simulink model "NewKitchen_REB_workstation"  (R2020b)
settings: Solver=FixedStepAuto  StartTime=sim_start  StopTime=sim_end  FixedStep=sim_interval  RelTol=1e-3
undefined symbols (not defined in the file): AmbientTem, Power1, Power2, Power3, Velocity1, Velocity2
libraries: dspswit3 x6
(part 2 of 3)

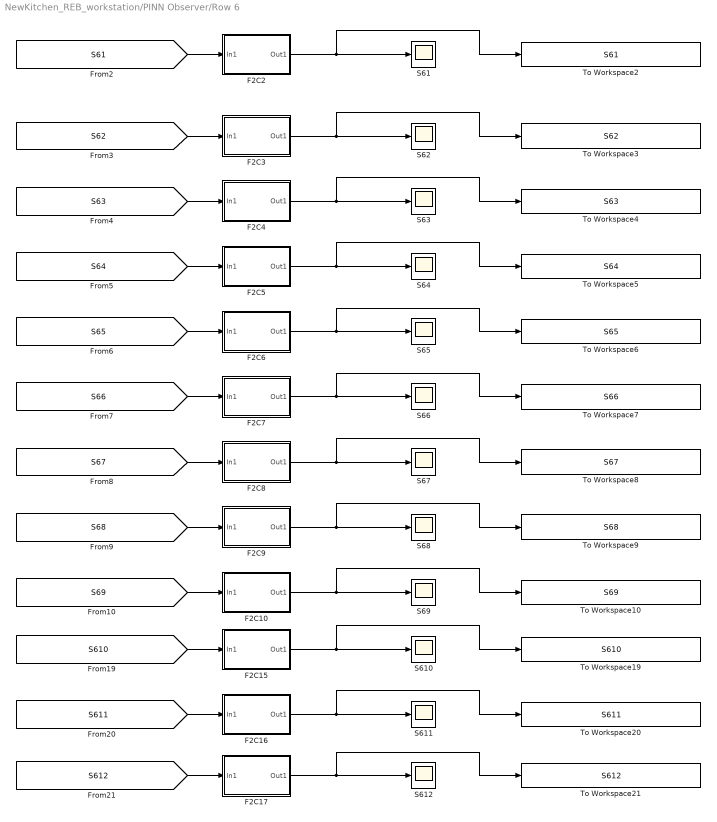
== system NewKitchen_REB_workstation/PINN Observer/Row 6 ==
  F2C10 : Subsystem
  F2C15 : Subsystem
  F2C16 : Subsystem
  F2C17 : Subsystem
  F2C2 : Subsystem
  F2C3 : Subsystem
  F2C4 : Subsystem
  F2C5 : Subsystem
  F2C6 : Subsystem
  F2C7 : Subsystem
  F2C8 : Subsystem
  F2C9 : Subsystem
  S{61..69,610..612} (12 alike) : Scope
  To Workspace10 : ToWorkspace  VariableName=S69  SampleTime=-1
  To Workspace19 : ToWorkspace  VariableName=S610  SampleTime=-1
  To Workspace2 : ToWorkspace  VariableName=S61  SampleTime=-1
  To Workspace20 : ToWorkspace  VariableName=S611  SampleTime=-1
  To Workspace21 : ToWorkspace  VariableName=S612  SampleTime=-1
  To Workspace3 : ToWorkspace  VariableName=S62  SampleTime=-1
  To Workspace4 : ToWorkspace  VariableName=S63  SampleTime=-1
  To Workspace5 : ToWorkspace  VariableName=S64  SampleTime=-1
  To Workspace6 : ToWorkspace  VariableName=S65  SampleTime=-1
  To Workspace7 : ToWorkspace  VariableName=S66  SampleTime=-1
  To Workspace8 : ToWorkspace  VariableName=S67  SampleTime=-1
  To Workspace9 : ToWorkspace  VariableName=S68  SampleTime=-1
  wires:
  [S64] -> F2C5/1(In1)
  [S62] -> F2C3/1(In1)
  [S63] -> F2C4/1(In1)
  F2C8/1(Out1) -> To Workspace8/1, S67/1
  F2C3/1(Out1) -> S62/1, To Workspace3/1
  F2C2/1(Out1) -> To Workspace2/1, S61/1
  [S61] -> F2C2/1(In1)
  F2C15/1(Out1) -> S610/1, To Workspace19/1
  [S68] -> F2C9/1(In1)
  [S611] -> F2C16/1(In1)
  F2C10/1(Out1) -> To Workspace10/1, S69/1
  F2C16/1(Out1) -> To Workspace20/1, S611/1
  F2C6/1(Out1) -> To Workspace6/1, S65/1
  [S610] -> F2C15/1(In1)
  F2C9/1(Out1) -> S68/1, To Workspace9/1
  [S66] -> F2C7/1(In1)
  F2C5/1(Out1) -> S64/1, To Workspace5/1
  F2C4/1(Out1) -> To Workspace4/1, S63/1
  [S612] -> F2C17/1(In1)
  [S65] -> F2C6/1(In1)
  F2C17/1(Out1) -> S612/1, To Workspace21/1
  F2C7/1(Out1) -> S66/1, To Workspace7/1
  [S69] -> F2C10/1(In1)
  [S67] -> F2C8/1(In1)

== system NewKitchen_REB_workstation/PINN Observer/Row 7 ==
  F2C10 : Subsystem
  F2C15 : Subsystem
  F2C16 : Subsystem
  F2C17 : Subsystem
  F2C2 : Subsystem
  F2C3 : Subsystem
  F2C4 : Subsystem
  F2C5 : Subsystem
  F2C6 : Subsystem
  F2C7 : Subsystem
  F2C8 : Subsystem
  F2C9 : Subsystem
  S{71..79,710..712} (12 alike) : Scope
  To Workspace10 : ToWorkspace  VariableName=S79  SampleTime=-1
  To Workspace19 : ToWorkspace  VariableName=S710  SampleTime=-1
  To Workspace2 : ToWorkspace  VariableName=S71  SampleTime=-1
  To Workspace20 : ToWorkspace  VariableName=S711  SampleTime=-1
  To Workspace21 : ToWorkspace  VariableName=S712  SampleTime=-1
  To Workspace3 : ToWorkspace  VariableName=S72  SampleTime=-1
  To Workspace4 : ToWorkspace  VariableName=S73  SampleTime=-1
  To Workspace5 : ToWorkspace  VariableName=S74  SampleTime=-1
  To Workspace6 : ToWorkspace  VariableName=S75  SampleTime=-1
  To Workspace7 : ToWorkspace  VariableName=S76  SampleTime=-1
  To Workspace8 : ToWorkspace  VariableName=S77  SampleTime=-1
  To Workspace9 : ToWorkspace  VariableName=S78  SampleTime=-1
  wires:
  [S77] -> F2C8/1(In1)
  [S79] -> F2C10/1(In1)
  F2C7/1(Out1) -> To Workspace7/1, S76/1
  F2C17/1(Out1) -> To Workspace21/1, S712/1
  [S75] -> F2C6/1(In1)
  [S712] -> F2C17/1(In1)
  F2C4/1(Out1) -> S73/1, To Workspace4/1
  F2C5/1(Out1) -> To Workspace5/1, S74/1
  [S76] -> F2C7/1(In1)
  F2C9/1(Out1) -> To Workspace9/1, S78/1
  [S710] -> F2C15/1(In1)
  F2C6/1(Out1) -> S75/1, To Workspace6/1
  F2C16/1(Out1) -> S711/1, To Workspace20/1
  F2C10/1(Out1) -> S79/1, To Workspace10/1
  [S711] -> F2C16/1(In1)
  [S78] -> F2C9/1(In1)
  F2C15/1(Out1) -> To Workspace19/1, S710/1
  [S71] -> F2C2/1(In1)
  F2C2/1(Out1) -> S71/1, To Workspace2/1
  F2C3/1(Out1) -> To Workspace3/1, S72/1
  F2C8/1(Out1) -> S77/1, To Workspace8/1
  [S73] -> F2C4/1(In1)
  [S72] -> F2C3/1(In1)
  [S74] -> F2C5/1(In1)

== system NewKitchen_REB_workstation/PINN Observer/Row 8 ==
  F2C10 : Subsystem
  F2C15 : Subsystem
  F2C16 : Subsystem
  F2C17 : Subsystem
  F2C2 : Subsystem
  F2C3 : Subsystem
  F2C4 : Subsystem
  F2C5 : Subsystem
  F2C6 : Subsystem
  F2C7 : Subsystem
  F2C8 : Subsystem
  F2C9 : Subsystem
  S{81..89,810..812} (12 alike) : Scope
  To Workspace10 : ToWorkspace  VariableName=S89  SampleTime=-1
  To Workspace19 : ToWorkspace  VariableName=S810  SampleTime=-1
  To Workspace2 : ToWorkspace  VariableName=S81  SampleTime=-1
  To Workspace20 : ToWorkspace  VariableName=S811  SampleTime=-1
  To Workspace21 : ToWorkspace  VariableName=S812  SampleTime=-1
  To Workspace3 : ToWorkspace  VariableName=S82  SampleTime=-1
  To Workspace4 : ToWorkspace  VariableName=S83  SampleTime=-1
  To Workspace5 : ToWorkspace  VariableName=S84  SampleTime=-1
  To Workspace6 : ToWorkspace  VariableName=S85  SampleTime=-1
  To Workspace7 : ToWorkspace  VariableName=S86  SampleTime=-1
  To Workspace8 : ToWorkspace  VariableName=S87  SampleTime=-1
  To Workspace9 : ToWorkspace  VariableName=S88  SampleTime=-1
  wires:
  [S84] -> F2C5/1(In1)
  [S82] -> F2C3/1(In1)
  [S83] -> F2C4/1(In1)
  F2C8/1(Out1) -> To Workspace8/1, S87/1
  F2C3/1(Out1) -> S82/1, To Workspace3/1
  F2C2/1(Out1) -> To Workspace2/1, S81/1
  [S81] -> F2C2/1(In1)
  F2C15/1(Out1) -> S810/1, To Workspace19/1
  [S88] -> F2C9/1(In1)
  [S811] -> F2C16/1(In1)
  F2C10/1(Out1) -> To Workspace10/1, S89/1
  F2C16/1(Out1) -> To Workspace20/1, S811/1
  F2C6/1(Out1) -> To Workspace6/1, S85/1
  [S810] -> F2C15/1(In1)
  F2C9/1(Out1) -> S88/1, To Workspace9/1
  [S86] -> F2C7/1(In1)
  F2C5/1(Out1) -> S84/1, To Workspace5/1
  F2C4/1(Out1) -> To Workspace4/1, S83/1
  [S812] -> F2C17/1(In1)
  [S85] -> F2C6/1(In1)
  F2C17/1(Out1) -> S812/1, To Workspace21/1
  F2C7/1(Out1) -> S86/1, To Workspace7/1
  [S89] -> F2C10/1(In1)
  [S87] -> F2C8/1(In1)

== system NewKitchen_REB_workstation/PINN Observer/Row 9 ==
  F2C10 : Subsystem
  F2C15 : Subsystem
  F2C16 : Subsystem
  F2C17 : Subsystem
  F2C2 : Subsystem
  F2C3 : Subsystem
  F2C4 : Subsystem
  F2C5 : Subsystem
  F2C6 : Subsystem
  F2C7 : Subsystem
  F2C8 : Subsystem
  F2C9 : Subsystem
  S{91..99,910..912} (12 alike) : Scope
  To Workspace10 : ToWorkspace  VariableName=S99  SampleTime=-1
  To Workspace19 : ToWorkspace  VariableName=S910  SampleTime=-1
  To Workspace2 : ToWorkspace  VariableName=S91  SampleTime=-1
  To Workspace20 : ToWorkspace  VariableName=S911  SampleTime=-1
  To Workspace21 : ToWorkspace  VariableName=S912  SampleTime=-1
  To Workspace3 : ToWorkspace  VariableName=S92  SampleTime=-1
  To Workspace4 : ToWorkspace  VariableName=S93  SampleTime=-1
  To Workspace5 : ToWorkspace  VariableName=S94  SampleTime=-1
  To Workspace6 : ToWorkspace  VariableName=S95  SampleTime=-1
  To Workspace7 : ToWorkspace  VariableName=S96  SampleTime=-1
  To Workspace8 : ToWorkspace  VariableName=S97  SampleTime=-1
  To Workspace9 : ToWorkspace  VariableName=S98  SampleTime=-1
  wires:
  [S97] -> F2C8/1(In1)
  [S99] -> F2C10/1(In1)
  F2C7/1(Out1) -> To Workspace7/1, S96/1
  F2C17/1(Out1) -> To Workspace21/1, S912/1
  [S95] -> F2C6/1(In1)
  [S912] -> F2C17/1(In1)
  F2C4/1(Out1) -> S93/1, To Workspace4/1
  F2C5/1(Out1) -> To Workspace5/1, S94/1
  [S96] -> F2C7/1(In1)
  F2C9/1(Out1) -> To Workspace9/1, S98/1
  [S910] -> F2C15/1(In1)
  F2C6/1(Out1) -> S95/1, To Workspace6/1
  F2C16/1(Out1) -> S911/1, To Workspace20/1
  F2C10/1(Out1) -> S99/1, To Workspace10/1
  [S911] -> F2C16/1(In1)
  [S98] -> F2C9/1(In1)
  F2C15/1(Out1) -> To Workspace19/1, S910/1
  [S91] -> F2C2/1(In1)
  F2C2/1(Out1) -> S91/1, To Workspace2/1
  F2C3/1(Out1) -> To Workspace3/1, S92/1
  F2C8/1(Out1) -> S97/1, To Workspace8/1
  [S93] -> F2C4/1(In1)
  [S92] -> F2C3/1(In1)
  [S94] -> F2C5/1(In1)

== system NewKitchen_REB_workstation/Signals/AmbientTem ==
  1-D Lookup Table : Lookup_n-D  NumberOfTableDimensions=1  BreakpointsForDimension1=AmbientTem(:,1)  Table=AmbientTem(:,2)  InterpMethod=Flat  InternalRulePriority=Speed  RndMeth=Simplest  InputSameDT=on
  Counter : dspswit3/Counter  Direction=Up  CountEvent=Free running  CounterSize=User defined  MaxCount=480  InitialCount=1  Output=Count  HitValue=1  ResetInput=off  SamplesPerFrame=1  Ts=60  CntDtype=double  HitDtype=Logical
  MATLAB Function : MATLAB Function  Commented=on  TreatAsAtomicUnit=on
  signal : Outport
  wires:
  Counter/1 -> 1-D Lookup Table/1
  1-D Lookup Table/1 -> signal/1

== system NewKitchen_REB_workstation/Signals/C2F3 ==
  signal : Inport
  Constant : Constant  Value=273.15
  Subtract : Sum
  Tout : Outport
  wires:
  signal/1 -> Subtract/1
  Constant/1 -> Subtract/2
  Subtract/1 -> Tout/1

== system NewKitchen_REB_workstation/Signals/Power1 ==
  1-D Lookup Table : Lookup_n-D  NumberOfTableDimensions=1  BreakpointsForDimension1=Power1(:,1)  Table=Power1(:,2)  InterpMethod=Flat  InternalRulePriority=Speed  RndMeth=Simplest  InputSameDT=on
  Counter : dspswit3/Counter  Direction=Up  CountEvent=Free running  CounterSize=User defined  MaxCount=480  InitialCount=1  Output=Count  HitValue=1  ResetInput=off  SamplesPerFrame=1  Ts=60  CntDtype=double  HitDtype=Logical
  MATLAB Function : MATLAB Function  Commented=on  TreatAsAtomicUnit=on
  P1 : Outport
  wires:
  Counter/1 -> 1-D Lookup Table/1
  1-D Lookup Table/1 -> P1/1

== system NewKitchen_REB_workstation/Signals/Power2 ==
  1-D Lookup Table : Lookup_n-D  NumberOfTableDimensions=1  BreakpointsForDimension1=Power2(:,1)  Table=Power2(:,2)  InterpMethod=Flat  InternalRulePriority=Speed  RndMeth=Simplest  InputSameDT=on
  Counter : dspswit3/Counter  Direction=Up  CountEvent=Free running  CounterSize=User defined  MaxCount=480  InitialCount=1  Output=Count  HitValue=1  ResetInput=off  SamplesPerFrame=1  Ts=60  CntDtype=double  HitDtype=Logical
  MATLAB Function : MATLAB Function  Commented=on  TreatAsAtomicUnit=on
  P2 : Outport
  wires:
  Counter/1 -> 1-D Lookup Table/1
  1-D Lookup Table/1 -> P2/1

== system NewKitchen_REB_workstation/Signals/Power3 ==
  1-D Lookup Table : Lookup_n-D  NumberOfTableDimensions=1  BreakpointsForDimension1=Power3(:,1)  Table=Power3(:,2)  InterpMethod=Flat  InternalRulePriority=Speed  RndMeth=Simplest  InputSameDT=on
  Counter : dspswit3/Counter  Direction=Up  CountEvent=Free running  CounterSize=User defined  MaxCount=480  InitialCount=1  Output=Count  HitValue=1  ResetInput=off  SamplesPerFrame=1  Ts=60  CntDtype=double  HitDtype=Logical
  MATLAB Function : MATLAB Function  Commented=on  TreatAsAtomicUnit=on
  P3 : Outport
  wires:
  Counter/1 -> 1-D Lookup Table/1
  1-D Lookup Table/1 -> P3/1

== system NewKitchen_REB_workstation/Signals/V1 ==
  1-D Lookup Table : Lookup_n-D  NumberOfTableDimensions=1  BreakpointsForDimension1=Velocity1(:,1)  Table=Velocity1(:,2)  InterpMethod=Flat  InternalRulePriority=Speed  RndMeth=Simplest  InputSameDT=on
  Counter : dspswit3/Counter  Direction=Up  CountEvent=Free running  CounterSize=User defined  MaxCount=480  InitialCount=1  Output=Count  HitValue=1  ResetInput=off  SamplesPerFrame=1  Ts=60  CntDtype=double  HitDtype=Logical
  MATLAB Function : MATLAB Function  Commented=on  TreatAsAtomicUnit=on
  V1 : Outport
  wires:
  Counter/1 -> 1-D Lookup Table/1
  1-D Lookup Table/1 -> V1/1

== system NewKitchen_REB_workstation/Signals/V2 ==
  1-D Lookup Table : Lookup_n-D  NumberOfTableDimensions=1  BreakpointsForDimension1=Velocity2(:,1)  Table=Velocity2(:,2)  InterpMethod=Flat  InternalRulePriority=Speed  RndMeth=Simplest  InputSameDT=on
  Counter : dspswit3/Counter  Direction=Up  CountEvent=Free running  CounterSize=User defined  MaxCount=480  InitialCount=1  Output=Count  HitValue=1  ResetInput=off  SamplesPerFrame=1  Ts=60  CntDtype=double  HitDtype=Logical
  MATLAB Function : MATLAB Function  Commented=on  TreatAsAtomicUnit=on
  V2 : Outport
  wires:
  Counter/1 -> 1-D Lookup Table/1
  1-D Lookup Table/1 -> V2/1

== system NewKitchen_REB_workstation/PINN Observer/Boundary Four/F2C10 ==
  In1 : Inport
  Constant : Constant  Value=273.15
  Subtract : Sum  Inputs=+-
  Out1 : Outport
  wires:
  In1/1 -> Subtract/1
  Constant/1 -> Subtract/2
  Subtract/1 -> Out1/1

== system NewKitchen_REB_workstation/PINN Observer/Boundary Four/F2C15 ==
  In1 : Inport
  Constant : Constant  Value=273.15
  Subtract : Sum  Inputs=+-
  Out1 : Outport
  wires:
  Subtract/1 -> Out1/1
  Constant/1 -> Subtract/2
  In1/1 -> Subtract/1

== system NewKitchen_REB_workstation/PINN Observer/Boundary Four/F2C16 ==
  In1 : Inport
  Constant : Constant  Value=273.15
  Subtract : Sum  Inputs=+-
  Out1 : Outport
  wires:
  In1/1 -> Subtract/1
  Constant/1 -> Subtract/2
  Subtract/1 -> Out1/1

== system NewKitchen_REB_workstation/PINN Observer/Boundary Four/F2C17 ==
  In1 : Inport
  Constant : Constant  Value=273.15
  Subtract : Sum  Inputs=+-
  Out1 : Outport
  wires:
  Subtract/1 -> Out1/1
  Constant/1 -> Subtract/2
  In1/1 -> Subtract/1

== system NewKitchen_REB_workstation/PINN Observer/Boundary Four/F2C18 ==
  In1 : Inport
  Constant : Constant  Value=273.15
  Subtract : Sum  Inputs=+-
  Out1 : Outport
  wires:
  In1/1 -> Subtract/1
  Constant/1 -> Subtract/2
  Subtract/1 -> Out1/1

== system NewKitchen_REB_workstation/PINN Observer/Boundary Four/F2C19 ==
  In1 : Inport
  Constant : Constant  Value=273.15
  Subtract : Sum  Inputs=+-
  Out1 : Outport
  wires:
  Subtract/1 -> Out1/1
  Constant/1 -> Subtract/2
  In1/1 -> Subtract/1

== system NewKitchen_REB_workstation/PINN Observer/Boundary Four/F2C2 ==
  In1 : Inport
  Constant : Constant  Value=273.15
  Subtract : Sum  Inputs=+-
  Out1 : Outport
  wires:
  In1/1 -> Subtract/1
  Constant/1 -> Subtract/2
  Subtract/1 -> Out1/1

== system NewKitchen_REB_workstation/PINN Observer/Boundary Four/F2C3 ==
  In1 : Inport
  Constant : Constant  Value=273.15
  Subtract : Sum  Inputs=+-
  Out1 : Outport
  wires:
  Subtract/1 -> Out1/1
  Constant/1 -> Subtract/2
  In1/1 -> Subtract/1

== system NewKitchen_REB_workstation/PINN Observer/Boundary Four/F2C4 ==
  In1 : Inport
  Constant : Constant  Value=273.15
  Subtract : Sum  Inputs=+-
  Out1 : Outport
  wires:
  In1/1 -> Subtract/1
  Constant/1 -> Subtract/2
  Subtract/1 -> Out1/1

== system NewKitchen_REB_workstation/PINN Observer/Boundary Four/F2C5 ==
  In1 : Inport
  Constant : Constant  Value=273.15
  Subtract : Sum  Inputs=+-
  Out1 : Outport
  wires:
  Subtract/1 -> Out1/1
  Constant/1 -> Subtract/2
  In1/1 -> Subtract/1

== system NewKitchen_REB_workstation/PINN Observer/Boundary Four/F2C6 ==
  In1 : Inport
  Constant : Constant  Value=273.15
  Subtract : Sum  Inputs=+-
  Out1 : Outport
  wires:
  In1/1 -> Subtract/1
  Constant/1 -> Subtract/2
  Subtract/1 -> Out1/1

== system NewKitchen_REB_workstation/PINN Observer/Boundary Four/F2C7 ==
  In1 : Inport
  Constant : Constant  Value=273.15
  Subtract : Sum  Inputs=+-
  Out1 : Outport
  wires:
  Subtract/1 -> Out1/1
  Constant/1 -> Subtract/2
  In1/1 -> Subtract/1

== system NewKitchen_REB_workstation/PINN Observer/Boundary Four/F2C8 ==
  In1 : Inport
  Constant : Constant  Value=273.15
  Subtract : Sum  Inputs=+-
  Out1 : Outport
  wires:
  In1/1 -> Subtract/1
  Constant/1 -> Subtract/2
  Subtract/1 -> Out1/1

== system NewKitchen_REB_workstation/PINN Observer/Boundary Four/F2C9 ==
  In1 : Inport
  Constant : Constant  Value=273.15
  Subtract : Sum  Inputs=+-
  Out1 : Outport
  wires:
  Subtract/1 -> Out1/1
  Constant/1 -> Subtract/2
  In1/1 -> Subtract/1

== system NewKitchen_REB_workstation/PINN Observer/Boundary One/F2C10 ==
  In1 : Inport
  Constant : Constant  Value=273.15
  Subtract : Sum  Inputs=+-
  Out1 : Outport
  wires:
  Subtract/1 -> Out1/1
  Constant/1 -> Subtract/2
  In1/1 -> Subtract/1

== system NewKitchen_REB_workstation/PINN Observer/Boundary One/F2C15 ==
  In1 : Inport
  Constant : Constant  Value=273.15
  Subtract : Sum  Inputs=+-
  Out1 : Outport
  wires:
  In1/1 -> Subtract/1
  Constant/1 -> Subtract/2
  Subtract/1 -> Out1/1

== system NewKitchen_REB_workstation/PINN Observer/Boundary One/F2C16 ==
  In1 : Inport
  Constant : Constant  Value=273.15
  Subtract : Sum  Inputs=+-
  Out1 : Outport
  wires:
  Subtract/1 -> Out1/1
  Constant/1 -> Subtract/2
  In1/1 -> Subtract/1

== system NewKitchen_REB_workstation/PINN Observer/Boundary One/F2C17 ==
  In1 : Inport
  Constant : Constant  Value=273.15
  Subtract : Sum  Inputs=+-
  Out1 : Outport
  wires:
  In1/1 -> Subtract/1
  Constant/1 -> Subtract/2
  Subtract/1 -> Out1/1

== system NewKitchen_REB_workstation/PINN Observer/Boundary One/F2C18 ==
  In1 : Inport
  Constant : Constant  Value=273.15
  Subtract : Sum  Inputs=+-
  Out1 : Outport
  wires:
  Subtract/1 -> Out1/1
  Constant/1 -> Subtract/2
  In1/1 -> Subtract/1

== system NewKitchen_REB_workstation/PINN Observer/Boundary One/F2C19 ==
  In1 : Inport
  Constant : Constant  Value=273.15
  Subtract : Sum  Inputs=+-
  Out1 : Outport
  wires:
  In1/1 -> Subtract/1
  Constant/1 -> Subtract/2
  Subtract/1 -> Out1/1

== system NewKitchen_REB_workstation/PINN Observer/Boundary One/F2C2 ==
  In1 : Inport
  Constant : Constant  Value=273.15
  Subtract : Sum  Inputs=+-
  Out1 : Outport
  wires:
  Subtract/1 -> Out1/1
  Constant/1 -> Subtract/2
  In1/1 -> Subtract/1

== system NewKitchen_REB_workstation/PINN Observer/Boundary One/F2C3 ==
  In1 : Inport
  Constant : Constant  Value=273.15
  Subtract : Sum  Inputs=+-
  Out1 : Outport
  wires:
  In1/1 -> Subtract/1
  Constant/1 -> Subtract/2
  Subtract/1 -> Out1/1

== system NewKitchen_REB_workstation/PINN Observer/Boundary One/F2C4 ==
  In1 : Inport
  Constant : Constant  Value=273.15
  Subtract : Sum  Inputs=+-
  Out1 : Outport
  wires:
  Subtract/1 -> Out1/1
  Constant/1 -> Subtract/2
  In1/1 -> Subtract/1

== system NewKitchen_REB_workstation/PINN Observer/Boundary One/F2C5 ==
  In1 : Inport
  Constant : Constant  Value=273.15
  Subtract : Sum  Inputs=+-
  Out1 : Outport
  wires:
  In1/1 -> Subtract/1
  Constant/1 -> Subtract/2
  Subtract/1 -> Out1/1

== system NewKitchen_REB_workstation/PINN Observer/Boundary One/F2C6 ==
  In1 : Inport
  Constant : Constant  Value=273.15
  Subtract : Sum  Inputs=+-
  Out1 : Outport
  wires:
  Subtract/1 -> Out1/1
  Constant/1 -> Subtract/2
  In1/1 -> Subtract/1

== system NewKitchen_REB_workstation/PINN Observer/Boundary One/F2C7 ==
  In1 : Inport
  Constant : Constant  Value=273.15
  Subtract : Sum  Inputs=+-
  Out1 : Outport
  wires:
  In1/1 -> Subtract/1
  Constant/1 -> Subtract/2
  Subtract/1 -> Out1/1

== system NewKitchen_REB_workstation/PINN Observer/Boundary One/F2C8 ==
  In1 : Inport
  Constant : Constant  Value=273.15
  Subtract : Sum  Inputs=+-
  Out1 : Outport
  wires:
  Subtract/1 -> Out1/1
  Constant/1 -> Subtract/2
  In1/1 -> Subtract/1

== system NewKitchen_REB_workstation/PINN Observer/Boundary One/F2C9 ==
  In1 : Inport
  Constant : Constant  Value=273.15
  Subtract : Sum  Inputs=+-
  Out1 : Outport
  wires:
  In1/1 -> Subtract/1
  Constant/1 -> Subtract/2
  Subtract/1 -> Out1/1

== system NewKitchen_REB_workstation/PINN Observer/Boundary Three/F2C10 ==
  In1 : Inport
  Constant : Constant  Value=273.15
  Subtract : Sum  Inputs=+-
  Out1 : Outport
  wires:
  Subtract/1 -> Out1/1
  Constant/1 -> Subtract/2
  In1/1 -> Subtract/1

== system NewKitchen_REB_workstation/PINN Observer/Boundary Three/F2C2 ==
  In1 : Inport
  Constant : Constant  Value=273.15
  Subtract : Sum  Inputs=+-
  Out1 : Outport
  wires:
  Subtract/1 -> Out1/1
  Constant/1 -> Subtract/2
  In1/1 -> Subtract/1

== system NewKitchen_REB_workstation/PINN Observer/Boundary Three/F2C3 ==
  In1 : Inport
  Constant : Constant  Value=273.15
  Subtract : Sum  Inputs=+-
  Out1 : Outport
  wires:
  In1/1 -> Subtract/1
  Constant/1 -> Subtract/2
  Subtract/1 -> Out1/1

== system NewKitchen_REB_workstation/PINN Observer/Boundary Three/F2C4 ==
  In1 : Inport
  Constant : Constant  Value=273.15
  Subtract : Sum  Inputs=+-
  Out1 : Outport
  wires:
  Subtract/1 -> Out1/1
  Constant/1 -> Subtract/2
  In1/1 -> Subtract/1

== system NewKitchen_REB_workstation/PINN Observer/Boundary Three/F2C5 ==
  In1 : Inport
  Constant : Constant  Value=273.15
  Subtract : Sum  Inputs=+-
  Out1 : Outport
  wires:
  In1/1 -> Subtract/1
  Constant/1 -> Subtract/2
  Subtract/1 -> Out1/1

== system NewKitchen_REB_workstation/PINN Observer/Boundary Three/F2C6 ==
  In1 : Inport
  Constant : Constant  Value=273.15
  Subtract : Sum  Inputs=+-
  Out1 : Outport
  wires:
  Subtract/1 -> Out1/1
  Constant/1 -> Subtract/2
  In1/1 -> Subtract/1

== system NewKitchen_REB_workstation/PINN Observer/Boundary Three/F2C7 ==
  In1 : Inport
  Constant : Constant  Value=273.15
  Subtract : Sum  Inputs=+-
  Out1 : Outport
  wires:
  In1/1 -> Subtract/1
  Constant/1 -> Subtract/2
  Subtract/1 -> Out1/1

== system NewKitchen_REB_workstation/PINN Observer/Boundary Three/F2C8 ==
  In1 : Inport
  Constant : Constant  Value=273.15
  Subtract : Sum  Inputs=+-
  Out1 : Outport
  wires:
  Subtract/1 -> Out1/1
  Constant/1 -> Subtract/2
  In1/1 -> Subtract/1

== system NewKitchen_REB_workstation/PINN Observer/Boundary Three/F2C9 ==
  In1 : Inport
  Constant : Constant  Value=273.15
  Subtract : Sum  Inputs=+-
  Out1 : Outport
  wires:
  In1/1 -> Subtract/1
  Constant/1 -> Subtract/2
  Subtract/1 -> Out1/1

== system NewKitchen_REB_workstation/PINN Observer/Boundary Two/F2C10 ==
  In1 : Inport
  Constant : Constant  Value=273.15
  Subtract : Sum  Inputs=+-
  Out1 : Outport
  wires:
  In1/1 -> Subtract/1
  Constant/1 -> Subtract/2
  Subtract/1 -> Out1/1

== system NewKitchen_REB_workstation/PINN Observer/Boundary Two/F2C2 ==
  In1 : Inport
  Constant : Constant  Value=273.15
  Subtract : Sum  Inputs=+-
  Out1 : Outport
  wires:
  In1/1 -> Subtract/1
  Constant/1 -> Subtract/2
  Subtract/1 -> Out1/1

== system NewKitchen_REB_workstation/PINN Observer/Boundary Two/F2C3 ==
  In1 : Inport
  Constant : Constant  Value=273.15
  Subtract : Sum  Inputs=+-
  Out1 : Outport
  wires:
  Subtract/1 -> Out1/1
  Constant/1 -> Subtract/2
  In1/1 -> Subtract/1

== system NewKitchen_REB_workstation/PINN Observer/Boundary Two/F2C4 ==
  In1 : Inport
  Constant : Constant  Value=273.15
  Subtract : Sum  Inputs=+-
  Out1 : Outport
  wires:
  In1/1 -> Subtract/1
  Constant/1 -> Subtract/2
  Subtract/1 -> Out1/1

== system NewKitchen_REB_workstation/PINN Observer/Boundary Two/F2C5 ==
  In1 : Inport
  Constant : Constant  Value=273.15
  Subtract : Sum  Inputs=+-
  Out1 : Outport
  wires:
  Subtract/1 -> Out1/1
  Constant/1 -> Subtract/2
  In1/1 -> Subtract/1

== system NewKitchen_REB_workstation/PINN Observer/Boundary Two/F2C6 ==
  In1 : Inport
  Constant : Constant  Value=273.15
  Subtract : Sum  Inputs=+-
  Out1 : Outport
  wires:
  In1/1 -> Subtract/1
  Constant/1 -> Subtract/2
  Subtract/1 -> Out1/1

== system NewKitchen_REB_workstation/PINN Observer/Boundary Two/F2C7 ==
  In1 : Inport
  Constant : Constant  Value=273.15
  Subtract : Sum  Inputs=+-
  Out1 : Outport
  wires:
  Subtract/1 -> Out1/1
  Constant/1 -> Subtract/2
  In1/1 -> Subtract/1

== system NewKitchen_REB_workstation/PINN Observer/Boundary Two/F2C8 ==
  In1 : Inport
  Constant : Constant  Value=273.15
  Subtract : Sum  Inputs=+-
  Out1 : Outport
  wires:
  In1/1 -> Subtract/1
  Constant/1 -> Subtract/2
  Subtract/1 -> Out1/1

== system NewKitchen_REB_workstation/PINN Observer/Boundary Two/F2C9 ==
  In1 : Inport
  Constant : Constant  Value=273.15
  Subtract : Sum  Inputs=+-
  Out1 : Outport
  wires:
  Subtract/1 -> Out1/1
  Constant/1 -> Subtract/2
  In1/1 -> Subtract/1

== system NewKitchen_REB_workstation/PINN Observer/Row 1/F2C10 ==
  In1 : Inport
  Constant : Constant  Value=273.15
  Subtract : Sum  Inputs=+-
  Out1 : Outport
  wires:
  Subtract/1 -> Out1/1
  Constant/1 -> Subtract/2
  In1/1 -> Subtract/1

== system NewKitchen_REB_workstation/PINN Observer/Row 1/F2C15 ==
  In1 : Inport
  Constant : Constant  Value=273.15
  Subtract : Sum  Inputs=+-
  Out1 : Outport
  wires:
  In1/1 -> Subtract/1
  Constant/1 -> Subtract/2
  Subtract/1 -> Out1/1

== system NewKitchen_REB_workstation/PINN Observer/Row 1/F2C16 ==
  In1 : Inport
  Constant : Constant  Value=273.15
  Subtract : Sum  Inputs=+-
  Out1 : Outport
  wires:
  Subtract/1 -> Out1/1
  Constant/1 -> Subtract/2
  In1/1 -> Subtract/1

== system NewKitchen_REB_workstation/PINN Observer/Row 1/F2C17 ==
  In1 : Inport
  Constant : Constant  Value=273.15
  Subtract : Sum  Inputs=+-
  Out1 : Outport
  wires:
  In1/1 -> Subtract/1
  Constant/1 -> Subtract/2
  Subtract/1 -> Out1/1

== system NewKitchen_REB_workstation/PINN Observer/Row 1/F2C2 ==
  In1 : Inport
  Constant : Constant  Value=273.15
  Subtract : Sum  Inputs=+-
  Out1 : Outport
  wires:
  Subtract/1 -> Out1/1
  Constant/1 -> Subtract/2
  In1/1 -> Subtract/1

== system NewKitchen_REB_workstation/PINN Observer/Row 1/F2C3 ==
  In1 : Inport
  Constant : Constant  Value=273.15
  Subtract : Sum  Inputs=+-
  Out1 : Outport
  wires:
  In1/1 -> Subtract/1
  Constant/1 -> Subtract/2
  Subtract/1 -> Out1/1

== system NewKitchen_REB_workstation/PINN Observer/Row 1/F2C4 ==
  In1 : Inport
  Constant : Constant  Value=273.15
  Subtract : Sum  Inputs=+-
  Out1 : Outport
  wires:
  Subtract/1 -> Out1/1
  Constant/1 -> Subtract/2
  In1/1 -> Subtract/1

== system NewKitchen_REB_workstation/PINN Observer/Row 1/F2C5 ==
  In1 : Inport
  Constant : Constant  Value=273.15
  Subtract : Sum  Inputs=+-
  Out1 : Outport
  wires:
  In1/1 -> Subtract/1
  Constant/1 -> Subtract/2
  Subtract/1 -> Out1/1

== system NewKitchen_REB_workstation/PINN Observer/Row 1/F2C6 ==
  In1 : Inport
  Constant : Constant  Value=273.15
  Subtract : Sum  Inputs=+-
  Out1 : Outport
  wires:
  Subtract/1 -> Out1/1
  Constant/1 -> Subtract/2
  In1/1 -> Subtract/1

== system NewKitchen_REB_workstation/PINN Observer/Row 1/F2C7 ==
  In1 : Inport
  Constant : Constant  Value=273.15
  Subtract : Sum  Inputs=+-
  Out1 : Outport
  wires:
  In1/1 -> Subtract/1
  Constant/1 -> Subtract/2
  Subtract/1 -> Out1/1

== system NewKitchen_REB_workstation/PINN Observer/Row 1/F2C8 ==
  In1 : Inport
  Constant : Constant  Value=273.15
  Subtract : Sum  Inputs=+-
  Out1 : Outport
  wires:
  Subtract/1 -> Out1/1
  Constant/1 -> Subtract/2
  In1/1 -> Subtract/1

== system NewKitchen_REB_workstation/PINN Observer/Row 1/F2C9 ==
  In1 : Inport
  Constant : Constant  Value=273.15
  Subtract : Sum  Inputs=+-
  Out1 : Outport
  wires:
  In1/1 -> Subtract/1
  Constant/1 -> Subtract/2
  Subtract/1 -> Out1/1

== system NewKitchen_REB_workstation/PINN Observer/Row 2/F2C10 ==
  In1 : Inport
  Constant : Constant  Value=273.15
  Subtract : Sum  Inputs=+-
  Out1 : Outport
  wires:
  In1/1 -> Subtract/1
  Constant/1 -> Subtract/2
  Subtract/1 -> Out1/1

== system NewKitchen_REB_workstation/PINN Observer/Row 2/F2C15 ==
  In1 : Inport
  Constant : Constant  Value=273.15
  Subtract : Sum  Inputs=+-
  Out1 : Outport
  wires:
  Subtract/1 -> Out1/1
  Constant/1 -> Subtract/2
  In1/1 -> Subtract/1

== system NewKitchen_REB_workstation/PINN Observer/Row 2/F2C16 ==
  In1 : Inport
  Constant : Constant  Value=273.15
  Subtract : Sum  Inputs=+-
  Out1 : Outport
  wires:
  In1/1 -> Subtract/1
  Constant/1 -> Subtract/2
  Subtract/1 -> Out1/1

== system NewKitchen_REB_workstation/PINN Observer/Row 2/F2C17 ==
  In1 : Inport
  Constant : Constant  Value=273.15
  Subtract : Sum  Inputs=+-
  Out1 : Outport
  wires:
  Subtract/1 -> Out1/1
  Constant/1 -> Subtract/2
  In1/1 -> Subtract/1

== system NewKitchen_REB_workstation/PINN Observer/Row 2/F2C2 ==
  In1 : Inport
  Constant : Constant  Value=273.15
  Subtract : Sum  Inputs=+-
  Out1 : Outport
  wires:
  In1/1 -> Subtract/1
  Constant/1 -> Subtract/2
  Subtract/1 -> Out1/1

== system NewKitchen_REB_workstation/PINN Observer/Row 2/F2C3 ==
  In1 : Inport
  Constant : Constant  Value=273.15
  Subtract : Sum  Inputs=+-
  Out1 : Outport
  wires:
  Subtract/1 -> Out1/1
  Constant/1 -> Subtract/2
  In1/1 -> Subtract/1

== system NewKitchen_REB_workstation/PINN Observer/Row 2/F2C4 ==
  In1 : Inport
  Constant : Constant  Value=273.15
  Subtract : Sum  Inputs=+-
  Out1 : Outport
  wires:
  In1/1 -> Subtract/1
  Constant/1 -> Subtract/2
  Subtract/1 -> Out1/1

== system NewKitchen_REB_workstation/PINN Observer/Row 2/F2C5 ==
  In1 : Inport
  Constant : Constant  Value=273.15
  Subtract : Sum  Inputs=+-
  Out1 : Outport
  wires:
  Subtract/1 -> Out1/1
  Constant/1 -> Subtract/2
  In1/1 -> Subtract/1

== system NewKitchen_REB_workstation/PINN Observer/Row 2/F2C6 ==
  In1 : Inport
  Constant : Constant  Value=273.15
  Subtract : Sum  Inputs=+-
  Out1 : Outport
  wires:
  In1/1 -> Subtract/1
  Constant/1 -> Subtract/2
  Subtract/1 -> Out1/1

== system NewKitchen_REB_workstation/PINN Observer/Row 2/F2C7 ==
  In1 : Inport
  Constant : Constant  Value=273.15
  Subtract : Sum  Inputs=+-
  Out1 : Outport
  wires:
  Subtract/1 -> Out1/1
  Constant/1 -> Subtract/2
  In1/1 -> Subtract/1

== system NewKitchen_REB_workstation/PINN Observer/Row 2/F2C8 ==
  In1 : Inport
  Constant : Constant  Value=273.15
  Subtract : Sum  Inputs=+-
  Out1 : Outport
  wires:
  In1/1 -> Subtract/1
  Constant/1 -> Subtract/2
  Subtract/1 -> Out1/1

== system NewKitchen_REB_workstation/PINN Observer/Row 2/F2C9 ==
  In1 : Inport
  Constant : Constant  Value=273.15
  Subtract : Sum  Inputs=+-
  Out1 : Outport
  wires:
  Subtract/1 -> Out1/1
  Constant/1 -> Subtract/2
  In1/1 -> Subtract/1

== system NewKitchen_REB_workstation/PINN Observer/Row 3/F2C10 ==
  In1 : Inport
  Constant : Constant  Value=273.15
  Subtract : Sum  Inputs=+-
  Out1 : Outport
  wires:
  Subtract/1 -> Out1/1
  Constant/1 -> Subtract/2
  In1/1 -> Subtract/1

== system NewKitchen_REB_workstation/PINN Observer/Row 3/F2C15 ==
  In1 : Inport
  Constant : Constant  Value=273.15
  Subtract : Sum  Inputs=+-
  Out1 : Outport
  wires:
  In1/1 -> Subtract/1
  Constant/1 -> Subtract/2
  Subtract/1 -> Out1/1

== system NewKitchen_REB_workstation/PINN Observer/Row 3/F2C16 ==
  In1 : Inport
  Constant : Constant  Value=273.15
  Subtract : Sum  Inputs=+-
  Out1 : Outport
  wires:
  Subtract/1 -> Out1/1
  Constant/1 -> Subtract/2
  In1/1 -> Subtract/1

== system NewKitchen_REB_workstation/PINN Observer/Row 3/F2C17 ==
  In1 : Inport
  Constant : Constant  Value=273.15
  Subtract : Sum  Inputs=+-
  Out1 : Outport
  wires:
  In1/1 -> Subtract/1
  Constant/1 -> Subtract/2
  Subtract/1 -> Out1/1

== system NewKitchen_REB_workstation/PINN Observer/Row 3/F2C2 ==
  In1 : Inport
  Constant : Constant  Value=273.15
  Subtract : Sum  Inputs=+-
  Out1 : Outport
  wires:
  Subtract/1 -> Out1/1
  Constant/1 -> Subtract/2
  In1/1 -> Subtract/1

== system NewKitchen_REB_workstation/PINN Observer/Row 3/F2C3 ==
  In1 : Inport
  Constant : Constant  Value=273.15
  Subtract : Sum  Inputs=+-
  Out1 : Outport
  wires:
  In1/1 -> Subtract/1
  Constant/1 -> Subtract/2
  Subtract/1 -> Out1/1

== system NewKitchen_REB_workstation/PINN Observer/Row 3/F2C4 ==
  In1 : Inport
  Constant : Constant  Value=273.15
  Subtract : Sum  Inputs=+-
  Out1 : Outport
  wires:
  Subtract/1 -> Out1/1
  Constant/1 -> Subtract/2
  In1/1 -> Subtract/1

== system NewKitchen_REB_workstation/PINN Observer/Row 3/F2C5 ==
  In1 : Inport
  Constant : Constant  Value=273.15
  Subtract : Sum  Inputs=+-
  Out1 : Outport
  wires:
  In1/1 -> Subtract/1
  Constant/1 -> Subtract/2
  Subtract/1 -> Out1/1

== system NewKitchen_REB_workstation/PINN Observer/Row 3/F2C6 ==
  In1 : Inport
  Constant : Constant  Value=273.15
  Subtract : Sum  Inputs=+-
  Out1 : Outport
  wires:
  Subtract/1 -> Out1/1
  Constant/1 -> Subtract/2
  In1/1 -> Subtract/1

== system NewKitchen_REB_workstation/PINN Observer/Row 3/F2C7 ==
  In1 : Inport
  Constant : Constant  Value=273.15
  Subtract : Sum  Inputs=+-
  Out1 : Outport
  wires:
  In1/1 -> Subtract/1
  Constant/1 -> Subtract/2
  Subtract/1 -> Out1/1

== system NewKitchen_REB_workstation/PINN Observer/Row 3/F2C8 ==
  In1 : Inport
  Constant : Constant  Value=273.15
  Subtract : Sum  Inputs=+-
  Out1 : Outport
  wires:
  Subtract/1 -> Out1/1
  Constant/1 -> Subtract/2
  In1/1 -> Subtract/1

== system NewKitchen_REB_workstation/PINN Observer/Row 3/F2C9 ==
  In1 : Inport
  Constant : Constant  Value=273.15
  Subtract : Sum  Inputs=+-
  Out1 : Outport
  wires:
  In1/1 -> Subtract/1
  Constant/1 -> Subtract/2
  Subtract/1 -> Out1/1

== system NewKitchen_REB_workstation/PINN Observer/Row 4/F2C10 ==
  In1 : Inport
  Constant : Constant  Value=273.15
  Subtract : Sum  Inputs=+-
  Out1 : Outport
  wires:
  In1/1 -> Subtract/1
  Constant/1 -> Subtract/2
  Subtract/1 -> Out1/1

== system NewKitchen_REB_workstation/PINN Observer/Row 4/F2C15 ==
  In1 : Inport
  Constant : Constant  Value=273.15
  Subtract : Sum  Inputs=+-
  Out1 : Outport
  wires:
  Subtract/1 -> Out1/1
  Constant/1 -> Subtract/2
  In1/1 -> Subtract/1

== system NewKitchen_REB_workstation/PINN Observer/Row 4/F2C16 ==
  In1 : Inport
  Constant : Constant  Value=273.15
  Subtract : Sum  Inputs=+-
  Out1 : Outport
  wires:
  In1/1 -> Subtract/1
  Constant/1 -> Subtract/2
  Subtract/1 -> Out1/1

== system NewKitchen_REB_workstation/PINN Observer/Row 4/F2C17 ==
  In1 : Inport
  Constant : Constant  Value=273.15
  Subtract : Sum  Inputs=+-
  Out1 : Outport
  wires:
  Subtract/1 -> Out1/1
  Constant/1 -> Subtract/2
  In1/1 -> Subtract/1

== system NewKitchen_REB_workstation/PINN Observer/Row 4/F2C2 ==
  In1 : Inport
  Constant : Constant  Value=273.15
  Subtract : Sum  Inputs=+-
  Out1 : Outport
  wires:
  In1/1 -> Subtract/1
  Constant/1 -> Subtract/2
  Subtract/1 -> Out1/1

== system NewKitchen_REB_workstation/PINN Observer/Row 4/F2C3 ==
  In1 : Inport
  Constant : Constant  Value=273.15
  Subtract : Sum  Inputs=+-
  Out1 : Outport
  wires:
  Subtract/1 -> Out1/1
  Constant/1 -> Subtract/2
  In1/1 -> Subtract/1

== system NewKitchen_REB_workstation/PINN Observer/Row 4/F2C4 ==
  In1 : Inport
  Constant : Constant  Value=273.15
  Subtract : Sum  Inputs=+-
  Out1 : Outport
  wires:
  In1/1 -> Subtract/1
  Constant/1 -> Subtract/2
  Subtract/1 -> Out1/1

== system NewKitchen_REB_workstation/PINN Observer/Row 4/F2C5 ==
  In1 : Inport
  Constant : Constant  Value=273.15
  Subtract : Sum  Inputs=+-
  Out1 : Outport
  wires:
  Subtract/1 -> Out1/1
  Constant/1 -> Subtract/2
  In1/1 -> Subtract/1

== system NewKitchen_REB_workstation/PINN Observer/Row 4/F2C6 ==
  In1 : Inport
  Constant : Constant  Value=273.15
  Subtract : Sum  Inputs=+-
  Out1 : Outport
  wires:
  In1/1 -> Subtract/1
  Constant/1 -> Subtract/2
  Subtract/1 -> Out1/1

== system NewKitchen_REB_workstation/PINN Observer/Row 4/F2C7 ==
  In1 : Inport
  Constant : Constant  Value=273.15
  Subtract : Sum  Inputs=+-
  Out1 : Outport
  wires:
  Subtract/1 -> Out1/1
  Constant/1 -> Subtract/2
  In1/1 -> Subtract/1

== system NewKitchen_REB_workstation/PINN Observer/Row 4/F2C8 ==
  In1 : Inport
  Constant : Constant  Value=273.15
  Subtract : Sum  Inputs=+-
  Out1 : Outport
  wires:
  In1/1 -> Subtract/1
  Constant/1 -> Subtract/2
  Subtract/1 -> Out1/1

== system NewKitchen_REB_workstation/PINN Observer/Row 4/F2C9 ==
  In1 : Inport
  Constant : Constant  Value=273.15
  Subtract : Sum  Inputs=+-
  Out1 : Outport
  wires:
  Subtract/1 -> Out1/1
  Constant/1 -> Subtract/2
  In1/1 -> Subtract/1

== system NewKitchen_REB_workstation/PINN Observer/Row 5/F2C10 ==
  In1 : Inport
  Constant : Constant  Value=273.15
  Subtract : Sum  Inputs=+-
  Out1 : Outport
  wires:
  Subtract/1 -> Out1/1
  Constant/1 -> Subtract/2
  In1/1 -> Subtract/1

== system NewKitchen_REB_workstation/PINN Observer/Row 5/F2C15 ==
  In1 : Inport
  Constant : Constant  Value=273.15
  Subtract : Sum  Inputs=+-
  Out1 : Outport
  wires:
  In1/1 -> Subtract/1
  Constant/1 -> Subtract/2
  Subtract/1 -> Out1/1

== system NewKitchen_REB_workstation/PINN Observer/Row 5/F2C16 ==
  In1 : Inport
  Constant : Constant  Value=273.15
  Subtract : Sum  Inputs=+-
  Out1 : Outport
  wires:
  Subtract/1 -> Out1/1
  Constant/1 -> Subtract/2
  In1/1 -> Subtract/1

== system NewKitchen_REB_workstation/PINN Observer/Row 5/F2C17 ==
  In1 : Inport
  Constant : Constant  Value=273.15
  Subtract : Sum  Inputs=+-
  Out1 : Outport
  wires:
  In1/1 -> Subtract/1
  Constant/1 -> Subtract/2
  Subtract/1 -> Out1/1

== system NewKitchen_REB_workstation/PINN Observer/Row 5/F2C2 ==
  In1 : Inport
  Constant : Constant  Value=273.15
  Subtract : Sum  Inputs=+-
  Out1 : Outport
  wires:
  Subtract/1 -> Out1/1
  Constant/1 -> Subtract/2
  In1/1 -> Subtract/1

== system NewKitchen_REB_workstation/PINN Observer/Row 5/F2C3 ==
  In1 : Inport
  Constant : Constant  Value=273.15
  Subtract : Sum  Inputs=+-
  Out1 : Outport
  wires:
  In1/1 -> Subtract/1
  Constant/1 -> Subtract/2
  Subtract/1 -> Out1/1

== system NewKitchen_REB_workstation/PINN Observer/Row 5/F2C4 ==
  In1 : Inport
  Constant : Constant  Value=273.15
  Subtract : Sum  Inputs=+-
  Out1 : Outport
  wires:
  Subtract/1 -> Out1/1
  Constant/1 -> Subtract/2
  In1/1 -> Subtract/1

== system NewKitchen_REB_workstation/PINN Observer/Row 5/F2C5 ==
  In1 : Inport
  Constant : Constant  Value=273.15
  Subtract : Sum  Inputs=+-
  Out1 : Outport
  wires:
  In1/1 -> Subtract/1
  Constant/1 -> Subtract/2
  Subtract/1 -> Out1/1

== system NewKitchen_REB_workstation/PINN Observer/Row 5/F2C6 ==
  In1 : Inport
  Constant : Constant  Value=273.15
  Subtract : Sum  Inputs=+-
  Out1 : Outport
  wires:
  Subtract/1 -> Out1/1
  Constant/1 -> Subtract/2
  In1/1 -> Subtract/1

== system NewKitchen_REB_workstation/PINN Observer/Row 5/F2C7 ==
  In1 : Inport
  Constant : Constant  Value=273.15
  Subtract : Sum  Inputs=+-
  Out1 : Outport
  wires:
  In1/1 -> Subtract/1
  Constant/1 -> Subtract/2
  Subtract/1 -> Out1/1

== system NewKitchen_REB_workstation/PINN Observer/Row 5/F2C8 ==
  In1 : Inport
  Constant : Constant  Value=273.15
  Subtract : Sum  Inputs=+-
  Out1 : Outport
  wires:
  Subtract/1 -> Out1/1
  Constant/1 -> Subtract/2
  In1/1 -> Subtract/1

== system NewKitchen_REB_workstation/PINN Observer/Row 5/F2C9 ==
  In1 : Inport
  Constant : Constant  Value=273.15
  Subtract : Sum  Inputs=+-
  Out1 : Outport
  wires:
  In1/1 -> Subtract/1
  Constant/1 -> Subtract/2
  Subtract/1 -> Out1/1

== system NewKitchen_REB_workstation/PINN Observer/Row 6/F2C10 ==
  In1 : Inport
  Constant : Constant  Value=273.15
  Subtract : Sum  Inputs=+-
  Out1 : Outport
  wires:
  In1/1 -> Subtract/1
  Constant/1 -> Subtract/2
  Subtract/1 -> Out1/1

== system NewKitchen_REB_workstation/PINN Observer/Row 6/F2C15 ==
  In1 : Inport
  Constant : Constant  Value=273.15
  Subtract : Sum  Inputs=+-
  Out1 : Outport
  wires:
  Subtract/1 -> Out1/1
  Constant/1 -> Subtract/2
  In1/1 -> Subtract/1

== system NewKitchen_REB_workstation/PINN Observer/Row 6/F2C16 ==
  In1 : Inport
  Constant : Constant  Value=273.15
  Subtract : Sum  Inputs=+-
  Out1 : Outport
  wires:
  In1/1 -> Subtract/1
  Constant/1 -> Subtract/2
  Subtract/1 -> Out1/1

== system NewKitchen_REB_workstation/PINN Observer/Row 6/F2C17 ==
  In1 : Inport
  Constant : Constant  Value=273.15
  Subtract : Sum  Inputs=+-
  Out1 : Outport
  wires:
  Subtract/1 -> Out1/1
  Constant/1 -> Subtract/2
  In1/1 -> Subtract/1

== system NewKitchen_REB_workstation/PINN Observer/Row 6/F2C2 ==
  In1 : Inport
  Constant : Constant  Value=273.15
  Subtract : Sum  Inputs=+-
  Out1 : Outport
  wires:
  In1/1 -> Subtract/1
  Constant/1 -> Subtract/2
  Subtract/1 -> Out1/1

== system NewKitchen_REB_workstation/PINN Observer/Row 6/F2C3 ==
  In1 : Inport
  Constant : Constant  Value=273.15
  Subtract : Sum  Inputs=+-
  Out1 : Outport
  wires:
  Subtract/1 -> Out1/1
  Constant/1 -> Subtract/2
  In1/1 -> Subtract/1

== system NewKitchen_REB_workstation/PINN Observer/Row 6/F2C4 ==
  In1 : Inport
  Constant : Constant  Value=273.15
  Subtract : Sum  Inputs=+-
  Out1 : Outport
  wires:
  In1/1 -> Subtract/1
  Constant/1 -> Subtract/2
  Subtract/1 -> Out1/1

== system NewKitchen_REB_workstation/PINN Observer/Row 6/F2C5 ==
  In1 : Inport
  Constant : Constant  Value=273.15
  Subtract : Sum  Inputs=+-
  Out1 : Outport
  wires:
  Subtract/1 -> Out1/1
  Constant/1 -> Subtract/2
  In1/1 -> Subtract/1

== system NewKitchen_REB_workstation/PINN Observer/Row 6/F2C6 ==
  In1 : Inport
  Constant : Constant  Value=273.15
  Subtract : Sum  Inputs=+-
  Out1 : Outport
  wires:
  In1/1 -> Subtract/1
  Constant/1 -> Subtract/2
  Subtract/1 -> Out1/1

== system NewKitchen_REB_workstation/PINN Observer/Row 6/F2C7 ==
  In1 : Inport
  Constant : Constant  Value=273.15
  Subtract : Sum  Inputs=+-
  Out1 : Outport
  wires:
  Subtract/1 -> Out1/1
  Constant/1 -> Subtract/2
  In1/1 -> Subtract/1

== system NewKitchen_REB_workstation/PINN Observer/Row 6/F2C8 ==
  In1 : Inport
  Constant : Constant  Value=273.15
  Subtract : Sum  Inputs=+-
  Out1 : Outport
  wires:
  In1/1 -> Subtract/1
  Constant/1 -> Subtract/2
  Subtract/1 -> Out1/1

== system NewKitchen_REB_workstation/PINN Observer/Row 6/F2C9 ==
  In1 : Inport
  Constant : Constant  Value=273.15
  Subtract : Sum  Inputs=+-
  Out1 : Outport
  wires:
  Subtract/1 -> Out1/1
  Constant/1 -> Subtract/2
  In1/1 -> Subtract/1

== system NewKitchen_REB_workstation/PINN Observer/Row 7/F2C10 ==
  In1 : Inport
  Constant : Constant  Value=273.15
  Subtract : Sum  Inputs=+-
  Out1 : Outport
  wires:
  Subtract/1 -> Out1/1
  Constant/1 -> Subtract/2
  In1/1 -> Subtract/1

== system NewKitchen_REB_workstation/PINN Observer/Row 7/F2C15 ==
  In1 : Inport
  Constant : Constant  Value=273.15
  Subtract : Sum  Inputs=+-
  Out1 : Outport
  wires:
  In1/1 -> Subtract/1
  Constant/1 -> Subtract/2
  Subtract/1 -> Out1/1

== system NewKitchen_REB_workstation/PINN Observer/Row 7/F2C16 ==
  In1 : Inport
  Constant : Constant  Value=273.15
  Subtract : Sum  Inputs=+-
  Out1 : Outport
  wires:
  Subtract/1 -> Out1/1
  Constant/1 -> Subtract/2
  In1/1 -> Subtract/1

== system NewKitchen_REB_workstation/PINN Observer/Row 7/F2C17 ==
  In1 : Inport
  Constant : Constant  Value=273.15
  Subtract : Sum  Inputs=+-
  Out1 : Outport
  wires:
  In1/1 -> Subtract/1
  Constant/1 -> Subtract/2
  Subtract/1 -> Out1/1

== system NewKitchen_REB_workstation/PINN Observer/Row 7/F2C2 ==
  In1 : Inport
  Constant : Constant  Value=273.15
  Subtract : Sum  Inputs=+-
  Out1 : Outport
  wires:
  Subtract/1 -> Out1/1
  Constant/1 -> Subtract/2
  In1/1 -> Subtract/1

== system NewKitchen_REB_workstation/PINN Observer/Row 7/F2C3 ==
  In1 : Inport
  Constant : Constant  Value=273.15
  Subtract : Sum  Inputs=+-
  Out1 : Outport
  wires:
  In1/1 -> Subtract/1
  Constant/1 -> Subtract/2
  Subtract/1 -> Out1/1

== system NewKitchen_REB_workstation/PINN Observer/Row 7/F2C4 ==
  In1 : Inport
  Constant : Constant  Value=273.15
  Subtract : Sum  Inputs=+-
  Out1 : Outport
  wires:
  Subtract/1 -> Out1/1
  Constant/1 -> Subtract/2
  In1/1 -> Subtract/1

== system NewKitchen_REB_workstation/PINN Observer/Row 7/F2C5 ==
  In1 : Inport
  Constant : Constant  Value=273.15
  Subtract : Sum  Inputs=+-
  Out1 : Outport
  wires:
  In1/1 -> Subtract/1
  Constant/1 -> Subtract/2
  Subtract/1 -> Out1/1

== system NewKitchen_REB_workstation/PINN Observer/Row 7/F2C6 ==
  In1 : Inport
  Constant : Constant  Value=273.15
  Subtract : Sum  Inputs=+-
  Out1 : Outport
  wires:
  Subtract/1 -> Out1/1
  Constant/1 -> Subtract/2
  In1/1 -> Subtract/1

== system NewKitchen_REB_workstation/PINN Observer/Row 7/F2C7 ==
  In1 : Inport
  Constant : Constant  Value=273.15
  Subtract : Sum  Inputs=+-
  Out1 : Outport
  wires:
  In1/1 -> Subtract/1
  Constant/1 -> Subtract/2
  Subtract/1 -> Out1/1

== system NewKitchen_REB_workstation/PINN Observer/Row 7/F2C8 ==
  In1 : Inport
  Constant : Constant  Value=273.15
  Subtract : Sum  Inputs=+-
  Out1 : Outport
  wires:
  Subtract/1 -> Out1/1
  Constant/1 -> Subtract/2
  In1/1 -> Subtract/1

== system NewKitchen_REB_workstation/PINN Observer/Row 7/F2C9 ==
  In1 : Inport
  Constant : Constant  Value=273.15
  Subtract : Sum  Inputs=+-
  Out1 : Outport
  wires:
  In1/1 -> Subtract/1
  Constant/1 -> Subtract/2
  Subtract/1 -> Out1/1

== system NewKitchen_REB_workstation/PINN Observer/Row 8/F2C10 ==
  In1 : Inport
  Constant : Constant  Value=273.15
  Subtract : Sum  Inputs=+-
  Out1 : Outport
  wires:
  In1/1 -> Subtract/1
  Constant/1 -> Subtract/2
  Subtract/1 -> Out1/1

== system NewKitchen_REB_workstation/PINN Observer/Row 8/F2C15 ==
  In1 : Inport
  Constant : Constant  Value=273.15
  Subtract : Sum  Inputs=+-
  Out1 : Outport
  wires:
  Subtract/1 -> Out1/1
  Constant/1 -> Subtract/2
  In1/1 -> Subtract/1

== system NewKitchen_REB_workstation/PINN Observer/Row 8/F2C16 ==
  In1 : Inport
  Constant : Constant  Value=273.15
  Subtract : Sum  Inputs=+-
  Out1 : Outport
  wires:
  In1/1 -> Subtract/1
  Constant/1 -> Subtract/2
  Subtract/1 -> Out1/1

== system NewKitchen_REB_workstation/PINN Observer/Row 8/F2C17 ==
  In1 : Inport
  Constant : Constant  Value=273.15
  Subtract : Sum  Inputs=+-
  Out1 : Outport
  wires:
  Subtract/1 -> Out1/1
  Constant/1 -> Subtract/2
  In1/1 -> Subtract/1

== system NewKitchen_REB_workstation/PINN Observer/Row 8/F2C2 ==
  In1 : Inport
  Constant : Constant  Value=273.15
  Subtract : Sum  Inputs=+-
  Out1 : Outport
  wires:
  In1/1 -> Subtract/1
  Constant/1 -> Subtract/2
  Subtract/1 -> Out1/1

== system NewKitchen_REB_workstation/PINN Observer/Row 8/F2C3 ==
  In1 : Inport
  Constant : Constant  Value=273.15
  Subtract : Sum  Inputs=+-
  Out1 : Outport
  wires:
  Subtract/1 -> Out1/1
  Constant/1 -> Subtract/2
  In1/1 -> Subtract/1

== system NewKitchen_REB_workstation/PINN Observer/Row 8/F2C4 ==
  In1 : Inport
  Constant : Constant  Value=273.15
  Subtract : Sum  Inputs=+-
  Out1 : Outport
  wires:
  In1/1 -> Subtract/1
  Constant/1 -> Subtract/2
  Subtract/1 -> Out1/1

== system NewKitchen_REB_workstation/PINN Observer/Row 8/F2C5 ==
  In1 : Inport
  Constant : Constant  Value=273.15
  Subtract : Sum  Inputs=+-
  Out1 : Outport
  wires:
  Subtract/1 -> Out1/1
  Constant/1 -> Subtract/2
  In1/1 -> Subtract/1

== system NewKitchen_REB_workstation/PINN Observer/Row 8/F2C6 ==
  In1 : Inport
  Constant : Constant  Value=273.15
  Subtract : Sum  Inputs=+-
  Out1 : Outport
  wires:
  In1/1 -> Subtract/1
  Constant/1 -> Subtract/2
  Subtract/1 -> Out1/1

== system NewKitchen_REB_workstation/PINN Observer/Row 8/F2C7 ==
  In1 : Inport
  Constant : Constant  Value=273.15
  Subtract : Sum  Inputs=+-
  Out1 : Outport
  wires:
  Subtract/1 -> Out1/1
  Constant/1 -> Subtract/2
  In1/1 -> Subtract/1

== system NewKitchen_REB_workstation/PINN Observer/Row 8/F2C8 ==
  In1 : Inport
  Constant : Constant  Value=273.15
  Subtract : Sum  Inputs=+-
  Out1 : Outport
  wires:
  In1/1 -> Subtract/1
  Constant/1 -> Subtract/2
  Subtract/1 -> Out1/1

== system NewKitchen_REB_workstation/PINN Observer/Row 8/F2C9 ==
  In1 : Inport
  Constant : Constant  Value=273.15
  Subtract : Sum  Inputs=+-
  Out1 : Outport
  wires:
  Subtract/1 -> Out1/1
  Constant/1 -> Subtract/2
  In1/1 -> Subtract/1

== system NewKitchen_REB_workstation/PINN Observer/Row 9/F2C10 ==
  In1 : Inport
  Constant : Constant  Value=273.15
  Subtract : Sum  Inputs=+-
  Out1 : Outport
  wires:
  Subtract/1 -> Out1/1
  Constant/1 -> Subtract/2
  In1/1 -> Subtract/1

== system NewKitchen_REB_workstation/PINN Observer/Row 9/F2C15 ==
  In1 : Inport
  Constant : Constant  Value=273.15
  Subtract : Sum  Inputs=+-
  Out1 : Outport
  wires:
  In1/1 -> Subtract/1
  Constant/1 -> Subtract/2
  Subtract/1 -> Out1/1

== system NewKitchen_REB_workstation/PINN Observer/Row 9/F2C16 ==
  In1 : Inport
  Constant : Constant  Value=273.15
  Subtract : Sum  Inputs=+-
  Out1 : Outport
  wires:
  Subtract/1 -> Out1/1
  Constant/1 -> Subtract/2
  In1/1 -> Subtract/1

== system NewKitchen_REB_workstation/PINN Observer/Row 9/F2C17 ==
  In1 : Inport
  Constant : Constant  Value=273.15
  Subtract : Sum  Inputs=+-
  Out1 : Outport
  wires:
  In1/1 -> Subtract/1
  Constant/1 -> Subtract/2
  Subtract/1 -> Out1/1

== system NewKitchen_REB_workstation/PINN Observer/Row 9/F2C2 ==
  In1 : Inport
  Constant : Constant  Value=273.15
  Subtract : Sum  Inputs=+-
  Out1 : Outport
  wires:
  Subtract/1 -> Out1/1
  Constant/1 -> Subtract/2
  In1/1 -> Subtract/1

== system NewKitchen_REB_workstation/PINN Observer/Row 9/F2C3 ==
  In1 : Inport
  Constant : Constant  Value=273.15
  Subtract : Sum  Inputs=+-
  Out1 : Outport
  wires:
  In1/1 -> Subtract/1
  Constant/1 -> Subtract/2
  Subtract/1 -> Out1/1

== system NewKitchen_REB_workstation/PINN Observer/Row 9/F2C4 ==
  In1 : Inport
  Constant : Constant  Value=273.15
  Subtract : Sum  Inputs=+-
  Out1 : Outport
  wires:
  Subtract/1 -> Out1/1
  Constant/1 -> Subtract/2
  In1/1 -> Subtract/1

== system NewKitchen_REB_workstation/PINN Observer/Row 9/F2C5 ==
  In1 : Inport
  Constant : Constant  Value=273.15
  Subtract : Sum  Inputs=+-
  Out1 : Outport
  wires:
  In1/1 -> Subtract/1
  Constant/1 -> Subtract/2
  Subtract/1 -> Out1/1

== system NewKitchen_REB_workstation/PINN Observer/Row 9/F2C6 ==
  In1 : Inport
  Constant : Constant  Value=273.15
  Subtract : Sum  Inputs=+-
  Out1 : Outport
  wires:
  Subtract/1 -> Out1/1
  Constant/1 -> Subtract/2
  In1/1 -> Subtract/1

== system NewKitchen_REB_workstation/PINN Observer/Row 9/F2C7 ==
  In1 : Inport
  Constant : Constant  Value=273.15
  Subtract : Sum  Inputs=+-
  Out1 : Outport
  wires:
  In1/1 -> Subtract/1
  Constant/1 -> Subtract/2
  Subtract/1 -> Out1/1

== system NewKitchen_REB_workstation/PINN Observer/Row 9/F2C8 ==
  In1 : Inport
  Constant : Constant  Value=273.15
  Subtract : Sum  Inputs=+-
  Out1 : Outport
  wires:
  Subtract/1 -> Out1/1
  Constant/1 -> Subtract/2
  In1/1 -> Subtract/1

== system NewKitchen_REB_workstation/PINN Observer/Row 9/F2C9 ==
  In1 : Inport
  Constant : Constant  Value=273.15
  Subtract : Sum  Inputs=+-
  Out1 : Outport
  wires:
  In1/1 -> Subtract/1
  Constant/1 -> Subtract/2
  Subtract/1 -> Out1/1
